simulink model "model_base_bros"  (R2017b)
settings: Solver=FixedStepDiscrete  StartTime=0.0  StopTime=inf  FixedStep=sampleTime  RelTol=1e-3
PostLoadFcn:
  | % load model parameters
  | % pname = fileparts(get_param('model_base_bros','filename'));
  | % run([pname  '\parameters_base_model_bros.m']);
  | parameters_base_model_bros;
  | 
  | % set requested state
  | set_param('model_base_bros/Requested state','Value',num2str(0));
InitFcn:
  | % load model parameters
  | % pname = fileparts(get_param('model_base_bros','filename'));
  | % run([pname  '\parameters_base_model_bros.m']);
  | parameters_base_model_bros;
  | 
  | % set requested state
  | set_param('model_base_bros/Requested state','Value',num2str(0));
StartFcn:
  | % load model parameters
  | % pname = fileparts(get_param('model_base_bros','filename'));
  | % run([pname  '\parameters_base_model_bros.m']);
  | parameters_base_model_bros;
  | 
  | % set requested state
  | set_param('model_base_bros/Requested state','Value',num2str(0));
StopFcn:
  | % switch off data logger (to hopefully avoid corrupt files). TwinCAT doesn't properly switch off the logger when shutting down the model
  | % no idea if this'll work.
  | set_param('model_base_bros/Record data (1 = yes, 0 = no)','Value',num2str(0));
values from neighbouring files (symbols this model uses):
  FFMatrix = -[0 -15; 15 0]    [parameters_base_model_bros.m]
  Lb = 0.07    [parameters_base_model_bros.m]
  Lf = 0.238    [parameters_base_model_bros.m]
  Lu = 0.153    [parameters_base_model_bros.m]
  msin_data_dist1 = [5 11 19 41 59 71 101 137 179 227 0.0358569687947 0.0275584886584 ... (30 elements, 10x3)]    [forcingfunction_data_id.mat]    (also in forcingfunction_data_id_2d_var6_1.mat = [0 0 0 0 0 0 0 0 0 0 0 0 ... (60 elements, 10x6)]; forcingfunction_data_id_2d_var75_nt11.mat = [0 0 0 0 0 0 0 0 0 0 0 0 ... (60 elements, 10x6)]; forcingfunction_data_id_nt10_var6.mat = [5 11 19 41 59 71 101 137 179 227 0.0248424367031 0.01909308)
  msin_data_dist2 = [7 13 23 43 61 73 103 139 181 229 0.0366642780879 0.0272817537998 ... (30 elements, 10x3)]    [forcingfunction_data_id.mat]    (also in forcingfunction_data_id_2d_var6_1.mat = [0 0 0 0 0 0 0 0 0 0 0 0 ... (60 elements, 10x6)]; forcingfunction_data_id_2d_var75_nt11.mat = [0 0 0 0 0 0 0 0 0 0 0 0 ... (60 elements, 10x6)]; forcingfunction_data_id_nt10_var6.mat = [7 13 23 43 61 73 103 139 181 229 0.0254017569884 0.01890135)
  msin_data_target = [2 9 17 27 37 47 0.0347382902327 0.0275101923829 0.0180185190239 0.0110214159229 0.0075682474126 0.00574660779142 ... (18 elements, 6x3)]    [forcingfunction_data_id.mat]    (also in forcingfunction_data_id_2d_var6_1.mat = [5 11 23 37 51 71 101 137 171 226 0.0252651788023 0.01941798; forcingfunction_data_id_2d_var75_nt11.mat = [5 11 23 37 51 71 101 137 173 227 263 0.0282088788597 ... (6; forcingfunction_data_id_nt10_var6.mat = [2 9 17 29 37 47 67 107 149 211 0.0239780224904 0.0189888450; forcingfunction_id_emg.mat = [3 7 13 19 31 0.0450441024419 0.0275859409824 0.015205627144)
  sampleTime = 0.001    [parameters_base_model_bros.m]
  Tm = 81.92    [forcingfunction_data_id_2d_var6_1.mat]    (also in forcingfunction_data_id_2d_var75_nt11.mat; forcingfunction_data_id_nt10_var6.mat; forcingfunction_id_emg.mat = 24)
undefined symbols (not defined in the file or in its folder): BROS1, BROS2, DiscIntNeverNeededParam
libraries: simulink x28, LibraryFM x14, VariousBlocksLibrary x13, simulink_extras x1
(part 2 of 4)

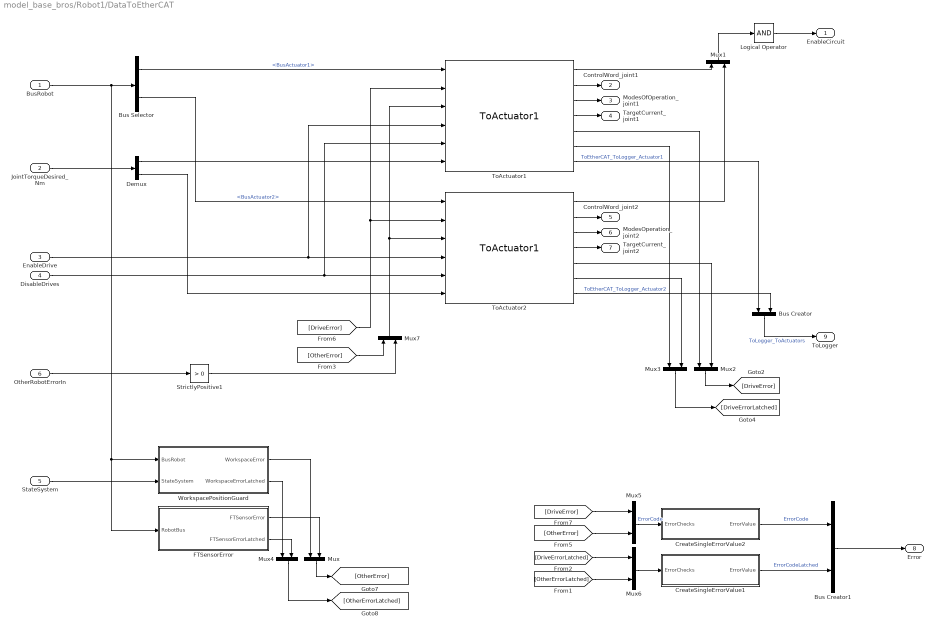
== system model_base_bros/Robot1/DataToEtherCAT ==
  BusRobot : Inport
  JointTorqueDesired_Nm : Inport  Port=2
  EnableDrive : Inport  Port=3
  DisableDrives : Inport  Port=4
  StateSystem : Inport  Port=5
  OtherRobotErrorIn : Inport  Port=6
  Bus Creator : BusCreator  Inputs=2
  Bus Creator1 : BusCreator  Inputs=2
  Bus Selector : BusSelector  OutputSignals=BusActuators.BusActuator1,BusActuators.BusActuator2
  CreateSingleErrorValue1 : Subsystem
  CreateSingleErrorValue2 : Subsystem
  Demux : Demux  Outputs=2
  FTSensorError : Subsystem
  Logical Operator : Logic  Inputs=1  AllPortsSameDT=off  OutDataTypeStr=boolean
  Mux{,1..7} (8 alike) : Mux  Inputs=2
  StrictlyPositive1 : simulink/Logic and Bit Operations/Compare To Zero  relop=>  OutDataTypeStr=boolean
  ToActuator1 : LibraryFM/ToActuator1  ActuatorStruct=RobotStruct.Actuator1
  ToActuator2 : LibraryFM/ToActuator1  ActuatorStruct=RobotStruct.Actuator2
  WorkspacePositionGuard : Subsystem
  EnableCircuit : Outport  OutDataTypeStr=boolean
  ControlWord_joint1 : Outport  Port=2  OutDataTypeStr=uint16
  ModesOfOperation_joint1 : Outport  Port=3  OutDataTypeStr=int8
  TargetCurrent_joint1 : Outport  Port=4  OutDataTypeStr=int16
  ControlWord_joint2 : Outport  Port=5  OutDataTypeStr=uint16
  ModesOperation_joint2 : Outport  Port=6  OutDataTypeStr=int8
  TargetCurrent_joint2 : Outport  Port=7  OutDataTypeStr=int16
  Error : Outport  Port=8
  ToLogger : Outport  Port=9
  wires:
  Bus Creator/1 -> ToLogger/1  "ToLogger_ToActuators"
  ToActuator2/7 -> Bus Creator/2  "ToEtherCAT_ToLogger_Actuator2"
  ToActuator1/7 -> Bus Creator/1  "ToEtherCAT_ToLogger_Actuator1"
  ToActuator1/5 -> Mux2/1
  ToActuator2/5 -> Mux2/2
  Mux2/1 -> [DriveError]
  ToActuator1/6 -> Mux3/1
  ToActuator2/6 -> Mux3/2
  [DriveError] -> ToActuator1/2, ToActuator2/2
  Mux1/1 -> Logical Operator/1
  ToActuator1/1 -> Mux1/1
  ToActuator2/1 -> Mux1/2
  ToActuator1/2 -> ControlWord_joint1/1
  ToActuator1/3 -> ModesOfOperation_joint1/1
  ToActuator2/2 -> ControlWord_joint2/1
  ToActuator1/4 -> TargetCurrent_joint1/1
  ToActuator2/4 -> TargetCurrent_joint2/1
  ToActuator2/3 -> ModesOperation_joint2/1
  Logical Operator/1 -> EnableCircuit/1
  Demux/2 -> ToActuator2/6
  JointTorqueDesired_Nm/1 -> Demux/1
  Demux/1 -> ToActuator1/6
  BusRobot/1 -> WorkspacePositionGuard/1(BusRobot), FTSensorError/1(RobotBus), Bus Selector/1
  Bus Selector/2 -> ToActuator2/1  "<BusActuator2>"
  Bus Selector/1 -> ToActuator1/1  "<BusActuator1>"
  DisableDrives/1 -> ToActuator1/5, ToActuator2/5
  EnableDrive/1 -> ToActuator1/4, ToActuator2/4
  Mux3/1 -> [DriveErrorLatched]
  StateSystem/1 -> WorkspacePositionGuard/2(StateSystem)
  FTSensorError/1(FTSensorError) -> Mux/2
  FTSensorError/2(FTSensorErrorLatched) -> Mux4/2
  WorkspacePositionGuard/1(WorkspaceError) -> Mux/1
  WorkspacePositionGuard/2(WorkspaceErrorLatched) -> Mux4/1
  Mux/1 -> [OtherError]
  Mux4/1 -> [OtherErrorLatched]
  [DriveError] -> Mux5/1
  [OtherError] -> Mux5/2
  CreateSingleErrorValue1/1(ErrorValue) -> Bus Creator1/2  "ErrorCodeLatched"
  [DriveErrorLatched] -> Mux6/1
  [OtherErrorLatched] -> Mux6/2
  Mux6/1 -> CreateSingleErrorValue1/1(ErrorChecks)
  Mux5/1 -> CreateSingleErrorValue2/1(ErrorChecks)  "ErrorCode"
  Bus Creator1/1 -> Error/1
  CreateSingleErrorValue2/1(ErrorValue) -> Bus Creator1/1  "ErrorCode"
  [OtherError] -> Mux7/1
  Mux7/1 -> ToActuator2/3, ToActuator1/3
  OtherRobotErrorIn/1 -> StrictlyPositive1/1
  StrictlyPositive1/1 -> Mux7/2

== system model_base_bros/Robot2/AppendToLoggerBus ==
  BusRobot : Inport
  ToEtherCAT_ToLogger : Inport  Port=2
  Controller_ToLogger : Inport  Port=3
  SystemState : Inport  Port=4
  Bus Creator : BusCreator  Inputs=8
  Bus Selector : BusSelector  OutputSignals=xOpSpace,qJointSpace,BusFTSensor,BusActuators
  Bus Selector1 : BusSelector  OutputSignals=ToEtherCAT_ToLogger_Actuator1,ToEtherCAT_ToLogger_Actuator2
  ToLogger : Outport
  wires:
  Bus Creator/1 -> ToLogger/1  "LoggerBus"
  Bus Selector/4 -> Bus Creator/4  "<BusActuators>"
  Bus Selector/1 -> Bus Creator/1  "<xOpSpace>"
  Bus Selector/3 -> Bus Creator/3  "<BusFTSensor>"
  Bus Selector/2 -> Bus Creator/2  "<qJointSpace>"
  BusRobot/1 -> Bus Selector/1
  ToEtherCAT_ToLogger/1 -> Bus Selector1/1
  Bus Selector1/1 -> Bus Creator/5  "<ToEtherCAT_ToLogger_Actuator1>"
  Bus Selector1/2 -> Bus Creator/6  "<ToEtherCAT_ToLogger_Actuator2>"
  Controller_ToLogger/1 -> Bus Creator/7
  SystemState/1 -> Bus Creator/8  "SystemState"

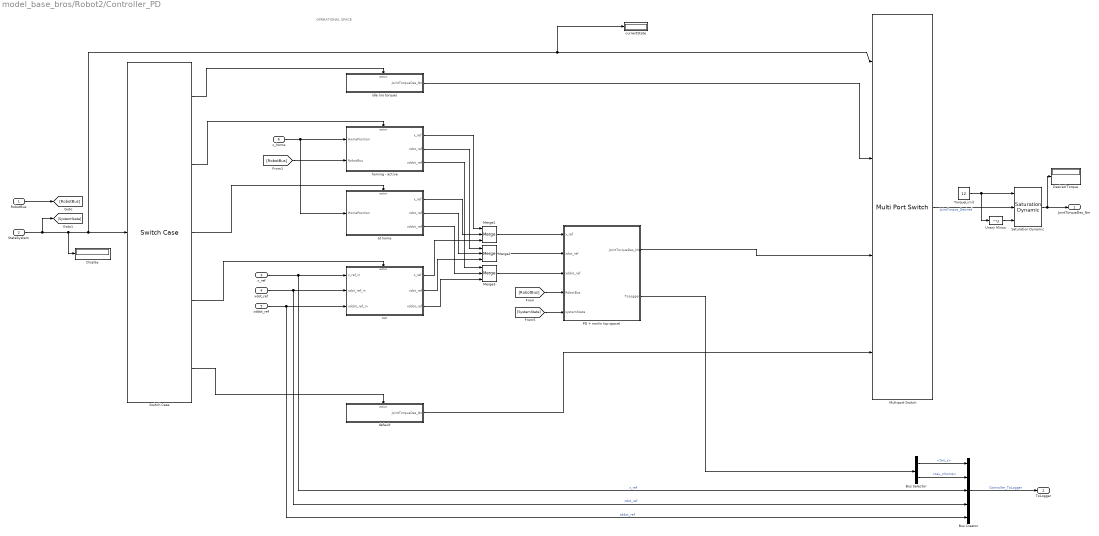
== system model_base_bros/Robot2/Controller_PD ==
  note: OPERATIONAL SPACE
  RobotBus : Inport
  StateSystem : Inport  Port=2
  x_ref : Inport  Port=3
  xdot_ref : Inport  Port=4
  xddot_ref : Inport  Port=5
  x_home : Inport  Port=6
  Bus Creator : BusCreator  Inputs=5
  Bus Selector : BusSelector  OutputSignals=tau_y,tau_nlcomp
  Desired Torque : Display
  Display : Display
  Merge1 : Merge  Inputs=3  InitialOutput=[0;0]
  Merge2 : Merge  Inputs=3  InitialOutput=[0;0]
  Merge3 : Merge  Inputs=3  InitialOutput=[0;0]
  Multiport Switch : MultiPortSwitch  DataPortOrder=Specify indices  Inputs=4  DataPortIndices={[0,1,2,201,299,301],[302,399,4]}  DataPortForDefault=Additional data port
  PD + nonlin (op space) : Subsystem
  Saturation Dynamic : simulink/Discontinuities/Saturation Dynamic  OutMin=[]  OutMax=[]  OutDataTypeStr=Inherit: Same as second input  OutDataType=fixdt(1, 16)  OutScaling=2^-10  DoSatur=off
  Switch Case : SwitchCase  CaseConditions={[0,1,2,201,299,301],302, 399,[4]}
  TorqueLimit : Constant  Value=12
  Unary Minus : UnaryMinus
  at home : Subsystem
  currentState : Display
  default : Subsystem  TreatAsAtomicUnit=on
  homing - active : Subsystem
  idle (no torque) : Subsystem  TreatAsAtomicUnit=on
  run : Subsystem
  JointTorqueDes_Nm : Outport
  ToLogger : Outport  Port=2
  wires:
  [SystemState] -> PD + nonlin (op space)/5(systemState)
  xddot_ref/1 -> Bus Creator/5, run/3(xddot_ref_in)  "xddot_ref"
  xdot_ref/1 -> Bus Creator/4, run/2(xdot_ref_in)  "xdot_ref"
  x_ref/1 -> Bus Creator/3, run/1(x_ref_in)  "x_ref"
  [RobotBus] -> PD + nonlin (op space)/4(RobotBus)
  RobotBus/1 -> [RobotBus]
  Merge3/1 -> PD + nonlin (op space)/3(xddot_ref)
  Merge2/1 -> PD + nonlin (op space)/2(xdot_ref)
  Merge1/1 -> PD + nonlin (op space)/1(x_ref)
  idle (no torque)/1(JointTorqueDes_Nm) -> Multiport Switch/2
  Switch Case/2 -> homing - active/Action
  Switch Case/1 -> idle (no torque)/Action
  default/1(JointTorqueDes_Nm) -> Multiport Switch/4
  Switch Case/5 -> default/Action
  Saturation Dynamic/1 -> Desired Torque/1, JointTorqueDes_Nm/1
  Switch Case/3 -> at home/Action
  homing - active/1(x_ref) -> Merge1/1
  run/1(x_ref) -> Merge1/3
  StateSystem/1 -> Display/1, Multiport Switch/1, currentState/1, Switch Case/1, [SystemState]
  run/2(xdot_ref) -> Merge2/3
  run/3(xddot_ref) -> Merge3/3
  homing - active/2(xdot_ref) -> Merge2/1
  homing - active/3(xddot_ref) -> Merge3/1
  Multiport Switch/1 -> Saturation Dynamic/2  "JointTorque_Desired"
  PD + nonlin (op space)/2(ToLogger) -> Bus Selector/1
  x_home/1 -> at home/1(HomePosition), homing - active/1(HomePosition)
  Bus Creator/1 -> ToLogger/1  "Controller_ToLogger"
  Bus Selector/1 -> Bus Creator/1  "<tau_y>"
  Bus Selector/2 -> Bus Creator/2  "<tau_nlcomp>"
  TorqueLimit/1 -> Unary Minus/1, Saturation Dynamic/1
  Unary Minus/1 -> Saturation Dynamic/3
  [RobotBus] -> homing - active/2(RobotBus)
  at home/1(x_ref) -> Merge1/2
  at home/2(xdot_ref) -> Merge2/2
  at home/3(xddot_ref) -> Merge3/2
  Switch Case/4 -> run/Action
  PD + nonlin (op space)/1(JointTorqueDes_Nm) -> Multiport Switch/3

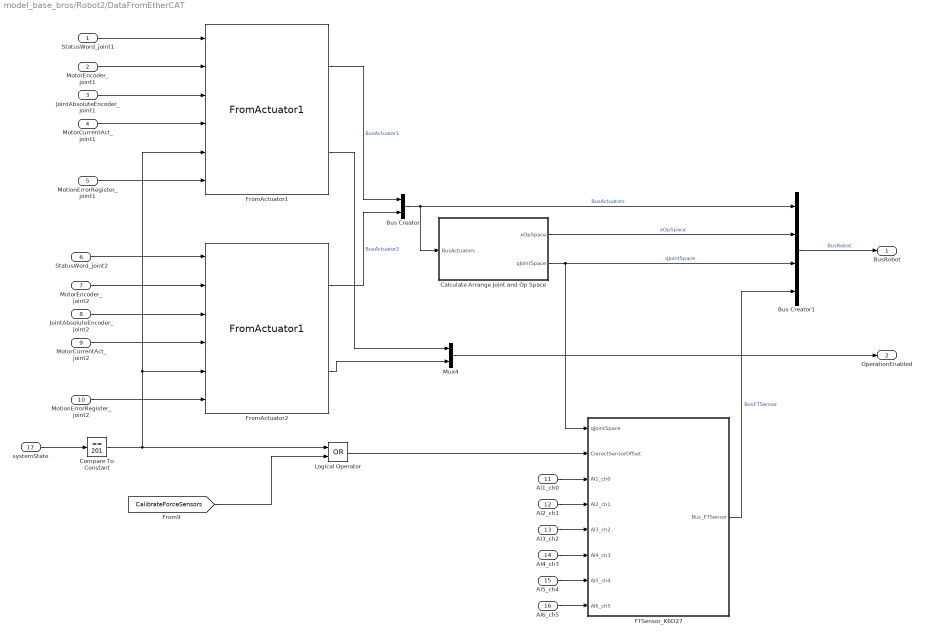
== system model_base_bros/Robot2/DataFromEtherCAT ==
  StatusWord_joint1 : Inport
  MotorEncoder_joint1 : Inport  Port=2
  JointAbsoluteEncoder_joint1 : Inport  Port=3
  MotorCurrentAct_joint1 : Inport  Port=4
  MotionErrorRegister_joint1 : Inport  Port=5  OutDataTypeStr=uint16
  StatusWord_joint2 : Inport  Port=6
  MotorEncoder_joint2 : Inport  Port=7
  "JointAbsoluteEncoder_joint2 " : Inport  Port=8
  MotorCurrentAct_joint2 : Inport  Port=9
  MotionErrorRegister_joint2 : Inport  Port=10  OutDataTypeStr=uint16
  AI1_ch0 : Inport  Port=11
  AI2_ch1 : Inport  Port=12
  AI3_ch2 : Inport  Port=13
  AI4_ch3 : Inport  Port=14
  AI5_ch4 : Inport  Port=15
  AI6_ch5 : Inport  Port=16
  systemState : Inport  Port=17
  Bus Creator : BusCreator  Inputs=2
  Bus Creator1 : BusCreator  Inputs=4
  Calculate Arrange Joint and Op Space : Subsystem
  Compare To Constant : simulink/Logic and Bit Operations/Compare To Constant  relop===  const=201  OutDataTypeStr=boolean
  FTSensor_K6D27 : Subsystem  mask{FTSensorStruct=RobotStruct.FTSensor}
      mask prompts: FTSensorStruct "Struct for force torque sensor"
  FromActuator1 : LibraryFM/FromActuator1  ActuatorStruct=RobotStruct.Actuator1
  FromActuator2 : LibraryFM/FromActuator1  ActuatorStruct=RobotStruct.Actuator2
  Logical Operator : Logic  Operator=OR  AllPortsSameDT=off  OutDataTypeStr=boolean
  Mux4 : Mux  Inputs=2
  BusRobot : Outport
  OperationEnabled : Outport  Port=2
  wires:
  FTSensor_K6D27/1(Bus_FTSensor) -> Bus Creator1/4  "BusFTSensor"
  FromActuator1/1 -> Bus Creator/1  "BusActuator1"
  FromActuator2/1 -> Bus Creator/2  "BusActuator2"
  FromActuator1/2 -> Mux4/1
  Mux4/1 -> OperationEnabled/1
  FromActuator2/2 -> Mux4/2
  MotorEncoder_joint1/1 -> FromActuator1/2
  StatusWord_joint1/1 -> FromActuator1/1
  JointAbsoluteEncoder_joint1/1 -> FromActuator1/3
  MotorCurrentAct_joint1/1 -> FromActuator1/4
  MotorEncoder_joint2/1 -> FromActuator2/2
  StatusWord_joint2/1 -> FromActuator2/1
  "JointAbsoluteEncoder_joint2 "/1 -> FromActuator2/3
  MotorCurrentAct_joint2/1 -> FromActuator2/4
  Bus Creator/1 -> Calculate Arrange Joint and Op Space/1(BusActuators), Bus Creator1/1  "BusActuators"
  Bus Creator1/1 -> BusRobot/1  "BusRobot"
  Calculate Arrange Joint and Op Space/2(qJointSpace) -> FTSensor_K6D27/1(qJointSpace), Bus Creator1/3  "qJointSpace"
  systemState/1 -> Compare To Constant/1
  AI1_ch0/1 -> FTSensor_K6D27/3(AI1_ch0)
  AI2_ch1/1 -> FTSensor_K6D27/4(AI2_ch1)
  AI3_ch2/1 -> FTSensor_K6D27/5(AI3_ch2)
  AI4_ch3/1 -> FTSensor_K6D27/6(AI4_ch3)
  AI5_ch4/1 -> FTSensor_K6D27/7(AI5_ch4)
  AI6_ch5/1 -> FTSensor_K6D27/8(AI6_ch5)
  Compare To Constant/1 -> Logical Operator/1, FromActuator1/5, FromActuator2/5
  Calculate Arrange Joint and Op Space/1(xOpSpace) -> Bus Creator1/2  "xOpSpace"
  [CalibrateForceSensors] -> Logical Operator/2
  Logical Operator/1 -> FTSensor_K6D27/2(CorrectSensorOffset)
  MotionErrorRegister_joint1/1 -> FromActuator1/6
  MotionErrorRegister_joint2/1 -> FromActuator2/6

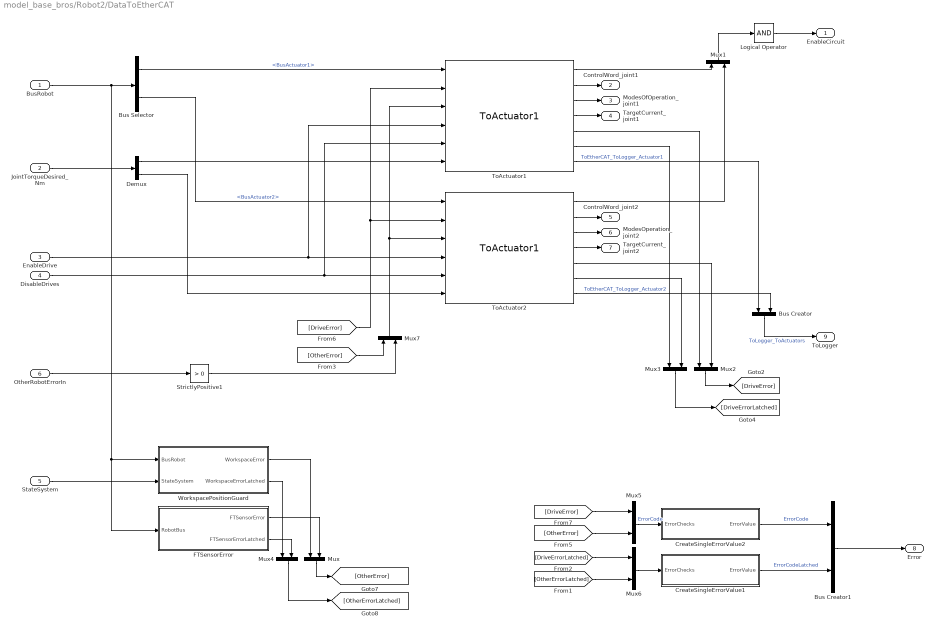
== system model_base_bros/Robot2/DataToEtherCAT ==
  BusRobot : Inport
  JointTorqueDesired_Nm : Inport  Port=2
  EnableDrive : Inport  Port=3
  DisableDrives : Inport  Port=4
  StateSystem : Inport  Port=5
  OtherRobotErrorIn : Inport  Port=6
  Bus Creator : BusCreator  Inputs=2
  Bus Creator1 : BusCreator  Inputs=2
  Bus Selector : BusSelector  OutputSignals=BusActuators.BusActuator1,BusActuators.BusActuator2
  CreateSingleErrorValue1 : Subsystem
  CreateSingleErrorValue2 : Subsystem
  Demux : Demux  Outputs=2
  FTSensorError : Subsystem
  Logical Operator : Logic  Inputs=1  AllPortsSameDT=off  OutDataTypeStr=boolean
  Mux{,1..7} (8 alike) : Mux  Inputs=2
  StrictlyPositive1 : simulink/Logic and Bit Operations/Compare To Zero  relop=>  OutDataTypeStr=boolean
  ToActuator1 : LibraryFM/ToActuator1  ActuatorStruct=RobotStruct.Actuator1
  ToActuator2 : LibraryFM/ToActuator1  ActuatorStruct=RobotStruct.Actuator2
  WorkspacePositionGuard : Subsystem
  EnableCircuit : Outport  OutDataTypeStr=boolean
  ControlWord_joint1 : Outport  Port=2  OutDataTypeStr=uint16
  ModesOfOperation_joint1 : Outport  Port=3  OutDataTypeStr=int8
  TargetCurrent_joint1 : Outport  Port=4  OutDataTypeStr=int16
  ControlWord_joint2 : Outport  Port=5  OutDataTypeStr=uint16
  ModesOperation_joint2 : Outport  Port=6  OutDataTypeStr=int8
  TargetCurrent_joint2 : Outport  Port=7  OutDataTypeStr=int16
  Error : Outport  Port=8
  ToLogger : Outport  Port=9
  wires:
  Bus Creator/1 -> ToLogger/1  "ToLogger_ToActuators"
  ToActuator2/7 -> Bus Creator/2  "ToEtherCAT_ToLogger_Actuator2"
  ToActuator1/7 -> Bus Creator/1  "ToEtherCAT_ToLogger_Actuator1"
  ToActuator1/5 -> Mux2/1
  ToActuator2/5 -> Mux2/2
  Mux2/1 -> [DriveError]
  ToActuator1/6 -> Mux3/1
  ToActuator2/6 -> Mux3/2
  [DriveError] -> ToActuator1/2, ToActuator2/2
  Mux1/1 -> Logical Operator/1
  ToActuator1/1 -> Mux1/1
  ToActuator2/1 -> Mux1/2
  ToActuator1/2 -> ControlWord_joint1/1
  ToActuator1/3 -> ModesOfOperation_joint1/1
  ToActuator2/2 -> ControlWord_joint2/1
  ToActuator1/4 -> TargetCurrent_joint1/1
  ToActuator2/4 -> TargetCurrent_joint2/1
  ToActuator2/3 -> ModesOperation_joint2/1
  Logical Operator/1 -> EnableCircuit/1
  Demux/2 -> ToActuator2/6
  JointTorqueDesired_Nm/1 -> Demux/1
  Demux/1 -> ToActuator1/6
  BusRobot/1 -> WorkspacePositionGuard/1(BusRobot), FTSensorError/1(RobotBus), Bus Selector/1
  Bus Selector/2 -> ToActuator2/1  "<BusActuator2>"
  Bus Selector/1 -> ToActuator1/1  "<BusActuator1>"
  DisableDrives/1 -> ToActuator1/5, ToActuator2/5
  EnableDrive/1 -> ToActuator1/4, ToActuator2/4
  Mux3/1 -> [DriveErrorLatched]
  StateSystem/1 -> WorkspacePositionGuard/2(StateSystem)
  FTSensorError/1(FTSensorError) -> Mux/2
  FTSensorError/2(FTSensorErrorLatched) -> Mux4/2
  WorkspacePositionGuard/1(WorkspaceError) -> Mux/1
  WorkspacePositionGuard/2(WorkspaceErrorLatched) -> Mux4/1
  Mux/1 -> [OtherError]
  Mux4/1 -> [OtherErrorLatched]
  [DriveError] -> Mux5/1
  [OtherError] -> Mux5/2
  CreateSingleErrorValue1/1(ErrorValue) -> Bus Creator1/2  "ErrorCodeLatched"
  [DriveErrorLatched] -> Mux6/1
  [OtherErrorLatched] -> Mux6/2
  Mux6/1 -> CreateSingleErrorValue1/1(ErrorChecks)
  Mux5/1 -> CreateSingleErrorValue2/1(ErrorChecks)  "ErrorCode"
  Bus Creator1/1 -> Error/1
  CreateSingleErrorValue2/1(ErrorValue) -> Bus Creator1/1  "ErrorCode"
  [OtherError] -> Mux7/1
  Mux7/1 -> ToActuator2/3, ToActuator1/3
  OtherRobotErrorIn/1 -> StrictlyPositive1/1
  StrictlyPositive1/1 -> Mux7/2

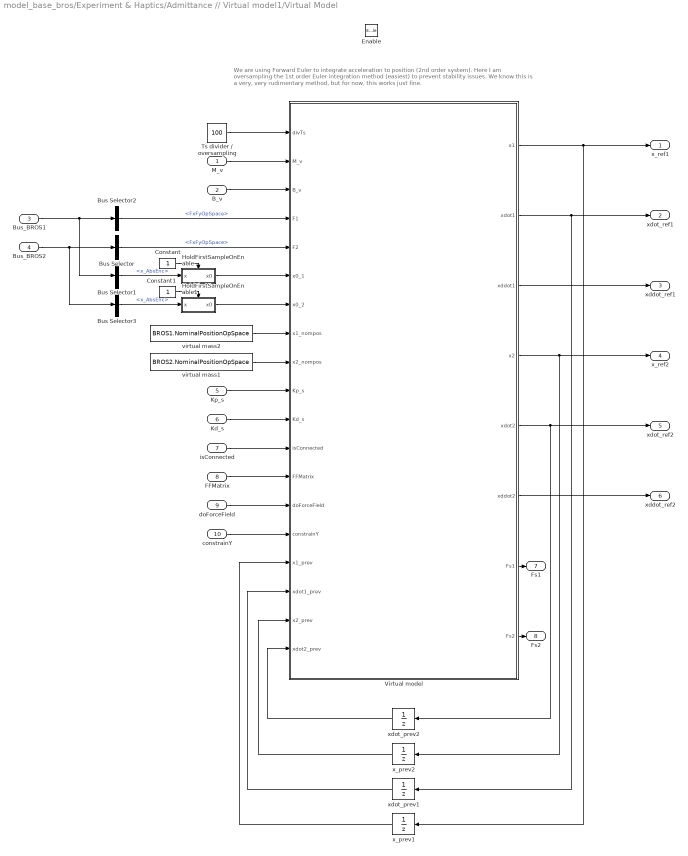
== system model_base_bros/Experiment & Haptics/Admittance // Virtual model1/Virtual Model ==
  note: We are using Forward Euler to integrate acceleration to position (2nd order system).
      | Here I am oversampling the 1st order Euler integration method (easiest) to prevent stability issues.
      | We know this is a very, very rudimentary method, but for now, this works just fine.
  M_v : Inport
  B_v : Inport  Port=2
  Bus_BROS1 : Inport  Port=3
  Bus_BROS2 : Inport  Port=4
  Kp_s : Inport  Port=5
  Kd_s : Inport  Port=6
  isConnected : Inport  Port=7
  FFMatrix : Inport  Port=8
  doForceField : Inport  Port=9
  constrainY : Inport  Port=10
  Enable : EnablePort  StatesWhenEnabling=reset
  Bus Selector : BusSelector  OutputSignals=BusFTSensor.FxFyOpSpace
  Bus Selector1 : BusSelector  OutputSignals=xOpSpace.x_AbsEnc
  Bus Selector2 : BusSelector  OutputSignals=BusFTSensor.FxFyOpSpace
  Bus Selector3 : BusSelector  OutputSignals=xOpSpace.x_AbsEnc
  Constant : Constant
  Constant1 : Constant
  HoldFirstSampleOnEnable : Subsystem
  HoldFirstSampleOnEnable1 : Subsystem
  Ts divider / oversampling : Constant  Value=100
  Virtual model : MATLAB Function  TreatAsAtomicUnit=on
  virtual mass1 : Constant  Value=BROS2.NominalPositionOpSpace
  virtual mass2 : Constant  Value=BROS1.NominalPositionOpSpace
  x_prev1 : UnitDelay  SampleTime=-1
  x_prev2 : UnitDelay  SampleTime=-1
  "xdot_prev1 " : UnitDelay  SampleTime=-1
  xdot_prev2 : UnitDelay  SampleTime=-1
  x_ref1 : Outport
  xdot_ref1 : Outport  Port=2
  xddot_ref1 : Outport  Port=3
  x_ref2 : Outport  Port=4
  xdot_ref2 : Outport  Port=5
  xddot_ref2 : Outport  Port=6
  Fs1 : Outport  Port=7
  Fs2 : Outport  Port=8
  wires:
  Constant/1 -> HoldFirstSampleOnEnable/Enable
  Bus Selector1/1 -> HoldFirstSampleOnEnable/1(x)  "<x_AbsEnc>"
  Bus Selector/1 -> Virtual model/5(F2)  "<FxFyOpSpace>"
  Virtual model/3(xddot1) -> xddot_ref1/1
  Virtual model/2(xdot1) -> xdot_ref1/1, "xdot_prev1 "/1
  HoldFirstSampleOnEnable1/1(x0) -> Virtual model/7(x0_2)
  Virtual model/4(x2) -> x_prev2/1, x_ref2/1
  x_prev1/1 -> Virtual model/16(x1_prev)
  virtual mass1/1 -> Virtual model/9(x2_nompos)
  virtual mass2/1 -> Virtual model/8(x1_nompos)
  Bus Selector2/1 -> Virtual model/4(F1)  "<FxFyOpSpace>"
  "xdot_prev1 "/1 -> Virtual model/17(xdot1_prev)
  isConnected/1 -> Virtual model/12(isConnected)
  x_prev2/1 -> Virtual model/18(x2_prev)
  Constant1/1 -> HoldFirstSampleOnEnable1/Enable
  Bus Selector3/1 -> HoldFirstSampleOnEnable1/1(x)  "<x_AbsEnc>"
  Kp_s/1 -> Virtual model/10(Kp_s)
  Kd_s/1 -> Virtual model/11(Kd_s)
  xdot_prev2/1 -> Virtual model/19(xdot2_prev)
  B_v/1 -> Virtual model/3(B_v)
  Bus_BROS1/1 -> Bus Selector2/1, Bus Selector1/1
  M_v/1 -> Virtual model/2(M_v)
  Bus_BROS2/1 -> Bus Selector3/1, Bus Selector/1
  HoldFirstSampleOnEnable/1(x0) -> Virtual model/6(x0_1)
  Virtual model/6(xddot2) -> xddot_ref2/1
  Virtual model/1(x1) -> x_ref1/1, x_prev1/1
  Virtual model/5(xdot2) -> xdot_prev2/1, xdot_ref2/1
  Ts divider / oversampling/1 -> Virtual model/1(divTs)
  doForceField/1 -> Virtual model/14(doForceField)
  FFMatrix/1 -> Virtual model/13(FFMatrix)
  Virtual model/7(Fs1) -> Fs1/1
  Virtual model/8(Fs2) -> Fs2/1
  constrainY/1 -> Virtual model/15(constrainY)

== system model_base_bros/Experiment & Haptics/Trial Logic/StopWatch ==
  Enable : EnablePort  StatesWhenEnabling=reset
  Counter Free-Running : simulink/Sources/Counter Free-Running  NumBits=32  tsamp=-1
  Data Type Conversion : DataTypeConversion  OutDataTypeStr=double
  sample time : Gain  Gain=sampleTime
  trialTime : Outport
  wires:
  sample time/1 -> trialTime/1
  Data Type Conversion/1 -> sample time/1
  Counter Free-Running/1 -> Data Type Conversion/1

== system model_base_bros/Robot1/Controller_PD/PD + nonlin (op space) ==
  x_ref : Inport
  xdot_ref : Inport  Port=2
  xddot_ref : Inport  Port=3
  RobotBus : Inport  Port=4
  systemState : Inport  Port=5
  Bus Creator : BusCreator  Inputs=2
  Bus Selector : BusSelector  OutputSignals=xOpSpace.x,xOpSpace.xdot,xOpSpace.x_AbsEnc,xOpSpace.xdot_AbsEnc,xOpSpace.J,xOpSpace.Jdot,qJointSpace.qdot_IncEnc
  DesiredTorque_PID : Display
  Gain : Gain  Gain=0
  Kd : Gain  Gain=15
  Kd1 : Gain  Gain=0
  Kd2 : Gain  Gain=5
  Kp : Gain  Gain=1500
  Sum{,2,4..5} (4 alike) : Sum  Inputs=|+-
  Sum1 : Sum  Inputs=|++
  Sum3 : Sum  Inputs=++++
  Terminator : Terminator
  Terminator1 : Terminator
  invJ1 : MATLAB Function  TreatAsAtomicUnit=on
  nonlinear compensation : MATLAB Function  TreatAsAtomicUnit=on
  JointTorqueDes_Nm : Outport
  ToLogger : Outport  Port=2
  wires:
  nonlinear compensation/1(tau) -> Gain/1, Bus Creator/2  "tau_nlcomp"
  invJ1/1(y) -> Sum1/1, Bus Creator/1  "tau_y"
  Bus Selector/1 -> Sum/2  "<x>"
  x_ref/1 -> Sum/1, Sum4/1  "q_ref"
  Sum/1 -> Kp/1  "e_p"
  xdot_ref/1 -> Sum5/1, Sum2/1  "qdot_ref"
  Sum2/1 -> Kd/1  "e_d"
  Sum1/1 -> JointTorqueDes_Nm/1, DesiredTorque_PID/1
  systemState/1 -> Terminator/1
  Bus Creator/1 -> ToLogger/1  "ToLoggerPD"
  Gain/1 -> Sum1/2
  Bus Selector/2 -> Sum2/2  "<xdot>"
  Bus Selector/6 -> nonlinear compensation/2(Jdot)  "<Jdot>"
  Bus Selector/5 -> nonlinear compensation/1(J), invJ1/2(J)  "<J>"
  RobotBus/1 -> Bus Selector/1
  Sum4/1 -> Kd1/1
  Sum5/1 -> Kd2/1
  xddot_ref/1 -> Terminator1/1  "qddot_ref"
  Bus Selector/3 -> Sum4/2  "<x_AbsEnc>"
  Bus Selector/4 -> Sum5/2  "<xdot_AbsEnc>"
  Kd/1 -> Sum3/2
  Kp/1 -> Sum3/1
  Sum3/1 -> invJ1/1(x)
  Kd1/1 -> Sum3/3
  Kd2/1 -> Sum3/4
  Bus Selector/7 -> nonlinear compensation/3(qdot)  "<qdot_IncEnc>"

== system model_base_bros/Robot1/Controller_PD/at home ==
  note: The velocity and acceleration references are set to [0;0] for stability.
  HomePosition : Inport
  Action Port : ActionPort  InitializeStates=reset  ActionType=case
  Constant : Constant
  Constant2 : Constant  Value=[0;0]
  Constant4 : Constant  Value=[0;0]
  HoldFirstSampleOnEnable : Subsystem
  x_ref : Outport  InitialOutput=[0;0]
  xdot_ref : Outport  Port=2  InitialOutput=[0;0]
  xddot_ref : Outport  Port=3  InitialOutput=[0;0]
  wires:
  Constant2/1 -> xdot_ref/1
  HoldFirstSampleOnEnable/1(x0) -> x_ref/1
  Constant4/1 -> xddot_ref/1
  Constant/1 -> HoldFirstSampleOnEnable/Enable
  HomePosition/1 -> HoldFirstSampleOnEnable/1(x)

== system model_base_bros/Robot1/Controller_PD/default ==
  Action Port : ActionPort  InitializeStates=reset  ActionType=default
  Constant3 : Constant  Value=[0;0]
  JointTorqueDes_Nm : Outport  InitialOutput=[0;0]
  wires:
  Constant3/1 -> JointTorqueDes_Nm/1

== system model_base_bros/Robot1/Controller_PD/homing - active ==
  note: The velocity and acceleration references are set to [0;0] for stability.
  HomePosition : Inport
  RobotBus : Inport  Port=2
  Action Port : ActionPort  InitializeStates=reset  ActionType=case
  Bus Selector : BusSelector  OutputSignals=xOpSpace.x
  Constant1 : Constant
  Constant2 : Constant  Value=[0;0]
  Constant4 : Constant  Value=[0;0]
  CrossFade : VariousBlocksLibrary/Various/CrossFade
  Cycloid : VariousBlocksLibrary/Various/Cycloid
  Rate Limiter : RateLimiter  RisingSlewLimit=0.1  FallingSlewLimit=-0.2  SampleTimeMode=inherited
  x_ref : Outport  InitialOutput=[0;0]
  xdot_ref : Outport  Port=2  InitialOutput=[0;0]
  xddot_ref : Outport  Port=3  InitialOutput=[0;0]
  wires:
  Constant2/1 -> xdot_ref/1
  Bus Selector/1 -> CrossFade/1  "<x>"
  RobotBus/1 -> Bus Selector/1
  HomePosition/1 -> CrossFade/2
  Cycloid/1 -> CrossFade/3
  Rate Limiter/1 -> Cycloid/1
  Constant1/1 -> Rate Limiter/1
  CrossFade/1 -> x_ref/1
  Constant4/1 -> xddot_ref/1

== system model_base_bros/Robot1/Controller_PD/idle (no torque) ==
  Action Port : ActionPort  InitializeStates=reset  ActionType=case
  Constant3 : Constant  Value=[0;0]
  JointTorqueDes_Nm : Outport  InitialOutput=[0;0]
  wires:
  Constant3/1 -> JointTorqueDes_Nm/1

== system model_base_bros/Robot1/Controller_PD/run ==
  x_ref_in : Inport
  xdot_ref_in : Inport  Port=2
  xddot_ref_in : Inport  Port=3
  Action Port : ActionPort  InitializeStates=reset  ActionType=case
  x_ref : Outport  InitialOutput=[0;0]
  xdot_ref : Outport  Port=2  InitialOutput=[0;0]
  xddot_ref : Outport  Port=3  InitialOutput=[0;0]
  wires:
  xdot_ref_in/1 -> xdot_ref/1
  xddot_ref_in/1 -> xddot_ref/1
  x_ref_in/1 -> x_ref/1

== system model_base_bros/Robot1/DataFromEtherCAT/Calculate Arrange Joint and Op Space ==
  note: Here all angles of the parallel mechanism are calculated
      | based on the endpoint position, though this may still lead to incorrect
      | estimations of the internal angles (e.g. it is possible that on of the elbows
      | has gone through a singular position already). So perhaps I should also include
      | a different way of calculating the internal angles
  BusActuators : Inport
  Bus Creator1 : BusCreator  Inputs=9
  Bus Creator2 : BusCreator  Inputs=6
  Bus Selector1 : BusSelector  OutputSignals=BusActuator1.JointPosition_AbsEnc_rad,BusActuator2.JointPosition_AbsEnc_rad,BusActuator1.JointVelocity_AbsEnc_rads,BusActuator2.JointVelocity_AbsEnc_rads
  Bus Selector2 : BusSelector  OutputSignals=BusActuator1.JointPosition_IncEnc_rad,BusActuator2.JointPosition_IncEnc_rad,BusActuator1.JointVelocity_IncEnc_rads,BusActuator2.JointVelocity_IncEnc_rads
  Bus Selector3 : BusSelector  OutputSignals=BusActuator1.JointTorque_Act_Nm,BusActuator2.JointTorque_Act_Nm
  Condition number : MATLAB Function  TreatAsAtomicUnit=on
  Ground : Ground
  Ground1 : Ground
  IK all joints : MATLAB Function  TreatAsAtomicUnit=on
  Mux{,1..4} (5 alike) : Mux  Inputs=2
  Terminator1 : Terminator
  Terminator2 : Terminator
  forward kinematics : Subsystem
  forward kinematics1 : Subsystem
  xOpSpace : Outport
  qJointSpace : Outport  Port=2
  wires:
  forward kinematics/5(Jdot) -> Bus Creator1/4  "Jdot"
  forward kinematics/3(xddot) -> Terminator1/1
  forward kinematics/2(xdot) -> Bus Creator1/2  "xdot"
  forward kinematics/1(x) -> IK all joints/1(x), Bus Creator1/1  "x"
  Bus Creator1/1 -> xOpSpace/1  "xOpSpace"
  forward kinematics/4(J) -> Condition number/1(J), Bus Creator1/3  "J"
  Ground/1 -> forward kinematics/3(JointAcceleration_rads2)
  Bus Creator2/1 -> qJointSpace/1  "qJointSpace"
  BusActuators/1 -> Bus Selector1/1, Bus Selector3/1, Bus Selector2/1
  Bus Selector2/1 -> Mux/1  "<JointPosition_IncEnc_rad>"
  Bus Selector2/2 -> Mux/2  "<JointPosition_IncEnc_rad>"
  Bus Selector2/3 -> Mux1/1  "<JointVelocity_IncEnc_rads>"
  Bus Selector2/4 -> Mux1/2  "<JointVelocity_IncEnc_rads>"
  Mux1/1 -> Bus Creator2/3, forward kinematics/2(JointVelocity_rads)  "qdot_IncEnc"
  Mux/1 -> forward kinematics/1(JointPosition_rad), Bus Creator2/2  "q_IncEnc"
  IK all joints/1(q_all) -> Bus Creator2/6  "q_all"
  Condition number/1(C) -> Bus Creator1/5  "conditioning"
  Bus Selector1/4 -> Mux3/2  "<JointVelocity_AbsEnc_rads>"
  Bus Selector1/3 -> Mux3/1  "<JointVelocity_AbsEnc_rads>"
  Bus Selector1/2 -> Mux2/2  "<JointPosition_AbsEnc_rad>"
  Bus Selector1/1 -> Mux2/1  "<JointPosition_AbsEnc_rad>"
  forward kinematics1/3(xddot) -> Terminator2/1
  Ground1/1 -> forward kinematics1/3(JointAcceleration_rads2)
  Mux2/1 -> Bus Creator2/4, forward kinematics1/1(JointPosition_rad)  "q_AbsEnc"
  Mux3/1 -> Bus Creator2/5, forward kinematics1/2(JointVelocity_rads)  "qdot_AbsEnc"
  forward kinematics1/2(xdot) -> Bus Creator1/7  "xdot_AbsEnc"
  forward kinematics1/1(x) -> Bus Creator1/6  "x_AbsEnc"
  forward kinematics1/4(J) -> Bus Creator1/8  "J_AbsEnc"
  forward kinematics1/5(Jdot) -> Bus Creator1/9  "Jdot_AbsEnc"
  Bus Selector3/1 -> Mux4/1  "<JointTorque_Act_Nm>"
  Bus Selector3/2 -> Mux4/2  "<JointTorque_Act_Nm>"
  Mux4/1 -> Bus Creator2/1  "JointTorque_Nm"

== system model_base_bros/Robot1/DataFromEtherCAT/FTSensor_K6D27 ==
  qJointSpace : Inport
  CorrectSensorOffset : Inport  Port=2
  AI1_ch0 : Inport  Port=3
  AI2_ch1 : Inport  Port=4
  AI3_ch2 : Inport  Port=5
  AI4_ch3 : Inport  Port=6
  AI5_ch4 : Inport  Port=7
  AI6_ch5 : Inport  Port=8
  Bus Creator : BusCreator  Inputs=3
  Bus Selector : BusSelector  OutputSignals=q_all
  Constant : Constant  Value=FTSensorStruct.TransformationMatrixSide
  CorrectOffset : MATLAB Function  TreatAsAtomicUnit=on
  Data Type Conversion{,1..5} (6 alike) : DataTypeConversion  OutDataTypeStr=double
  Detect Increase : simulink/Logic and Bit Operations/Detect Increase  vinit=0.0  InputProcessing=Inherited  OutDataTypeStr=boolean
  Mux : Mux  Inputs=6
  Selector : Selector  InputPortWidth=6  IndexOptions=Index vector (dialog)  Indices=[1 2]  OutputSizes=1
  SensorToOperationalSpace : MATLAB Function  TreatAsAtomicUnit=on
  Terminator : Terminator
  force (op space) : Display
  force (sensor space) : Display
  spikefilter : Subsystem
  Bus_FTSensor : Outport
  wires:
  Constant/1 -> SensorToOperationalSpace/3(transmatside)
  Bus Creator/1 -> Bus_FTSensor/1  "BusFTSensor"
  SensorToOperationalSpace/1(FTOpSpace) -> Selector/1, force (op space)/1, Bus Creator/1  "ForcesOpSpace"
  Data Type Conversion5/1 -> Mux/6
  Data Type Conversion4/1 -> Mux/5
  Data Type Conversion3/1 -> Mux/4
  Data Type Conversion2/1 -> Mux/3
  Data Type Conversion1/1 -> Mux/2
  Data Type Conversion/1 -> Mux/1
  CorrectOffset/1(u_out) -> spikefilter/1(in)  "ForcesSensorSpace"
  CorrectOffset/2(corrected) -> Terminator/1
  AI3_ch2/1 -> Data Type Conversion2/1
  AI4_ch3/1 -> Data Type Conversion3/1
  AI5_ch4/1 -> Data Type Conversion4/1
  AI6_ch5/1 -> Data Type Conversion5/1
  Detect Increase/1 -> CorrectOffset/2(reset)
  CorrectSensorOffset/1 -> Detect Increase/1
  Mux/1 -> CorrectOffset/1(u_in)
  AI1_ch0/1 -> Data Type Conversion/1
  AI2_ch1/1 -> Data Type Conversion1/1
  qJointSpace/1 -> Bus Selector/1
  Bus Selector/1 -> SensorToOperationalSpace/1(q_all)  "<q_all>"
  Selector/1 -> Bus Creator/2  "FxFyOpSpace"
  spikefilter/1(out) -> SensorToOperationalSpace/2(Fs), Bus Creator/3, force (sensor space)/1  "ForcesSensorSpace"

== system model_base_bros/Robot1/DataToEtherCAT/CreateSingleErrorValue1 ==
  ErrorChecks : Inport
  Data Type Conversion1 : DataTypeConversion  OutDataTypeStr=double
  ErrorToPower2 : MATLAB Function  TreatAsAtomicUnit=on
  ErrorValue : Outport
  wires:
  Data Type Conversion1/1 -> ErrorToPower2/1(u)
  ErrorChecks/1 -> Data Type Conversion1/1
  ErrorToPower2/1(e) -> ErrorValue/1

== system model_base_bros/Robot1/DataToEtherCAT/CreateSingleErrorValue2 ==
  ErrorChecks : Inport
  Data Type Conversion1 : DataTypeConversion  OutDataTypeStr=double
  ErrorToPower2 : MATLAB Function  TreatAsAtomicUnit=on
  ErrorValue : Outport
  wires:
  Data Type Conversion1/1 -> ErrorToPower2/1(u)
  ErrorChecks/1 -> Data Type Conversion1/1
  ErrorToPower2/1(e) -> ErrorValue/1

== system model_base_bros/Robot1/DataToEtherCAT/FTSensorError ==
  RobotBus : Inport
  AvoidAlgebraicLoop : Memory
  Bus Selector : BusSelector  OutputSignals=BusFTSensor.ForcesSensorSpace
  Constant : Constant  Value=RobotStruct.FTSensor.MaxAllowableForcesTorqueSensor
  Data Type Conversion1 : DataTypeConversion  OutDataTypeStr=boolean
  Detect Change : simulink/Logic and Bit Operations/Detect Change  vinit=0  InputProcessing=Inherited  OutDataTypeStr=boolean
  FTSensorLastError : Display
  LatchRising : LibraryFM/Utilities/LatchRising  ic=0
  MATLAB Function : MATLAB Function  TreatAsAtomicUnit=on
  ShowFTSensorErrorLatched : Display
  FTSensorError : Outport
  FTSensorErrorLatched : Outport  Port=2
  wires:
  Constant/1 -> MATLAB Function/2(MaxForcesTorques)
  MATLAB Function/1(e) -> Data Type Conversion1/1, FTSensorLastError/1
  LatchRising/1 -> ShowFTSensorErrorLatched/1, FTSensorErrorLatched/1
  AvoidAlgebraicLoop/1 -> Detect Change/1, LatchRising/1, FTSensorError/1
  Detect Change/1 -> LatchRising/Trigger
  RobotBus/1 -> Bus Selector/1
  Bus Selector/1 -> MATLAB Function/1(ForcesTorques)  "<ForcesSensorSpace>"
  Data Type Conversion1/1 -> AvoidAlgebraicLoop/1

== system model_base_bros/Robot1/DataToEtherCAT/WorkspacePositionGuard ==
  note: Check internal angles
  note: Check whether endpoint position is within the predefined workspace
      | (ellipse)
  note: Check for singularity of joint configuration by checking
      | the condition number. When it exceeds a certain value, go to a safe mode
      | For now, this means disabling the actuators.
      | Note that the boundaries set using admittance should prohibit this from happening.
      | However, if sometjhing really goes wrong, this is a safe guard
  BusRobot : Inport
  StateSystem : Inport  Port=2
  AvoidAlgebraicLoop : Memory
  Bus Selector : BusSelector  OutputSignals=xOpSpace.x,xOpSpace.conditioning,qJointSpace.q_all
  CheckInternalAngles : MATLAB Function  TreatAsAtomicUnit=on
  Compare To Constant : simulink/Logic and Bit Operations/Compare To Constant  relop=>  const=4  OutDataTypeStr=boolean
  Compare To Constant1 : simulink/Logic and Bit Operations/Compare To Constant  relop=>=  const=2.75  OutDataTypeStr=boolean
  Data Type Conversion1 : DataTypeConversion  OutDataTypeStr=boolean
  Data Type Conversion2 : DataTypeConversion  Commented=through  OutDataTypeStr=int32
  Data Type Conversion4 : DataTypeConversion  OutDataTypeStr=boolean
  Detect Change : simulink/Logic and Bit Operations/Detect Change  vinit=0  InputProcessing=Inherited  OutDataTypeStr=boolean
  EndpointPositionGuard : MATLAB Function  TreatAsAtomicUnit=on
  LatchRising : LibraryFM/Utilities/LatchRising  ic=0
  Logical Operator : Logic  Operator=OR  AllPortsSameDT=off  OutDataTypeStr=boolean
  Mux : Mux  Inputs=2
  ShowWorkspaceErrorLatched : Display
  WorkspaceLastError : Display
  WorkspaceError : Outport
  WorkspaceErrorLatched : Outport  Port=2
  wires:
  BusRobot/1 -> Bus Selector/1
  Bus Selector/1 -> EndpointPositionGuard/2(xe)  "<x>"
  LatchRising/1 -> Data Type Conversion2/1
  EndpointPositionGuard/1(error) -> Data Type Conversion1/1
  Mux/1 -> AvoidAlgebraicLoop/1, WorkspaceLastError/1
  Detect Change/1 -> LatchRising/Trigger
  AvoidAlgebraicLoop/1 -> WorkspaceError/1, Detect Change/1, LatchRising/1
  Compare To Constant/1 -> EndpointPositionGuard/1(correctState)
  Bus Selector/2 -> Compare To Constant1/1  "<conditioning>"
  StateSystem/1 -> Compare To Constant/1
  Data Type Conversion2/1 -> WorkspaceErrorLatched/1, ShowWorkspaceErrorLatched/1
  CheckInternalAngles/1(angleError) -> Data Type Conversion4/1
  Bus Selector/3 -> CheckInternalAngles/1(theta)  "<q_all>"
  Data Type Conversion4/1 -> Mux/2
  Logical Operator/1 -> Mux/1
  Data Type Conversion1/1 -> Logical Operator/1
  Compare To Constant1/1 -> Logical Operator/2

== system model_base_bros/Robot2/Controller_PD/PD + nonlin (op space) ==
  x_ref : Inport
  xdot_ref : Inport  Port=2
  xddot_ref : Inport  Port=3
  RobotBus : Inport  Port=4
  systemState : Inport  Port=5
  Bus Creator : BusCreator  Inputs=2
  Bus Selector : BusSelector  OutputSignals=xOpSpace.x,xOpSpace.xdot,xOpSpace.x_AbsEnc,xOpSpace.xdot_AbsEnc,xOpSpace.J,xOpSpace.Jdot,qJointSpace.qdot_IncEnc
  DesiredTorque_PID : Display
  Gain : Gain  Gain=0
  Kd : Gain  Gain=15
  Kd1 : Gain  Gain=0
  Kd2 : Gain  Gain=5
  Kp : Gain  Gain=1500
  Sum{,2,4..5} (4 alike) : Sum  Inputs=|+-
  Sum1 : Sum  Inputs=|++
  Sum3 : Sum  Inputs=++++
  Terminator : Terminator
  Terminator1 : Terminator
  invJ1 : MATLAB Function  TreatAsAtomicUnit=on
  nonlinear compensation : MATLAB Function  TreatAsAtomicUnit=on
  JointTorqueDes_Nm : Outport
  ToLogger : Outport  Port=2
  wires:
  nonlinear compensation/1(tau) -> Gain/1, Bus Creator/2  "tau_nlcomp"
  invJ1/1(y) -> Sum1/1, Bus Creator/1  "tau_y"
  Bus Selector/1 -> Sum/2  "<x>"
  x_ref/1 -> Sum/1, Sum4/1  "q_ref"
  Sum/1 -> Kp/1  "e_p"
  xdot_ref/1 -> Sum5/1, Sum2/1  "qdot_ref"
  Sum2/1 -> Kd/1  "e_d"
  Sum1/1 -> JointTorqueDes_Nm/1, DesiredTorque_PID/1
  systemState/1 -> Terminator/1
  Bus Creator/1 -> ToLogger/1  "ToLoggerPD"
  Gain/1 -> Sum1/2
  Bus Selector/2 -> Sum2/2  "<xdot>"
  Bus Selector/6 -> nonlinear compensation/2(Jdot)  "<Jdot>"
  Bus Selector/5 -> nonlinear compensation/1(J), invJ1/2(J)  "<J>"
  RobotBus/1 -> Bus Selector/1
  Sum4/1 -> Kd1/1
  Sum5/1 -> Kd2/1
  xddot_ref/1 -> Terminator1/1  "qddot_ref"
  Bus Selector/3 -> Sum4/2  "<x_AbsEnc>"
  Bus Selector/4 -> Sum5/2  "<xdot_AbsEnc>"
  Kd/1 -> Sum3/2
  Kp/1 -> Sum3/1
  Sum3/1 -> invJ1/1(x)
  Kd1/1 -> Sum3/3
  Kd2/1 -> Sum3/4
  Bus Selector/7 -> nonlinear compensation/3(qdot)  "<qdot_IncEnc>"

== system model_base_bros/Robot2/Controller_PD/at home ==
  note: The velocity and acceleration references are set to [0;0] for stability.
  HomePosition : Inport
  Action Port : ActionPort  InitializeStates=reset  ActionType=case
  Constant : Constant
  Constant2 : Constant  Value=[0;0]
  Constant4 : Constant  Value=[0;0]
  HoldFirstSampleOnEnable : Subsystem
  x_ref : Outport  InitialOutput=[0;0]
  xdot_ref : Outport  Port=2  InitialOutput=[0;0]
  xddot_ref : Outport  Port=3  InitialOutput=[0;0]
  wires:
  Constant2/1 -> xdot_ref/1
  HoldFirstSampleOnEnable/1(x0) -> x_ref/1
  Constant4/1 -> xddot_ref/1
  Constant/1 -> HoldFirstSampleOnEnable/Enable
  HomePosition/1 -> HoldFirstSampleOnEnable/1(x)

== system model_base_bros/Robot2/Controller_PD/default ==
  Action Port : ActionPort  InitializeStates=reset  ActionType=default
  Constant3 : Constant  Value=[0;0]
  JointTorqueDes_Nm : Outport  InitialOutput=[0;0]
  wires:
  Constant3/1 -> JointTorqueDes_Nm/1

== system model_base_bros/Robot2/Controller_PD/homing - active ==
  note: The velocity and acceleration references are set to [0;0] for stability.
  HomePosition : Inport
  RobotBus : Inport  Port=2
  Action Port : ActionPort  InitializeStates=reset  ActionType=case
  Bus Selector : BusSelector  OutputSignals=xOpSpace.x
  Constant1 : Constant
  Constant2 : Constant  Value=[0;0]
  Constant4 : Constant  Value=[0;0]
  CrossFade : VariousBlocksLibrary/Various/CrossFade
  Cycloid : VariousBlocksLibrary/Various/Cycloid
  Rate Limiter : RateLimiter  RisingSlewLimit=0.1  FallingSlewLimit=-0.2  SampleTimeMode=inherited
  x_ref : Outport  InitialOutput=[0;0]
  xdot_ref : Outport  Port=2  InitialOutput=[0;0]
  xddot_ref : Outport  Port=3  InitialOutput=[0;0]
  wires:
  Constant2/1 -> xdot_ref/1
  Bus Selector/1 -> CrossFade/1  "<x>"
  RobotBus/1 -> Bus Selector/1
  HomePosition/1 -> CrossFade/2
  Cycloid/1 -> CrossFade/3
  Rate Limiter/1 -> Cycloid/1
  Constant1/1 -> Rate Limiter/1
  CrossFade/1 -> x_ref/1
  Constant4/1 -> xddot_ref/1

== system model_base_bros/Robot2/Controller_PD/idle (no torque) ==
  Action Port : ActionPort  InitializeStates=reset  ActionType=case
  Constant3 : Constant  Value=[0;0]
  JointTorqueDes_Nm : Outport  InitialOutput=[0;0]
  wires:
  Constant3/1 -> JointTorqueDes_Nm/1

== system model_base_bros/Robot2/Controller_PD/run ==
  x_ref_in : Inport
  xdot_ref_in : Inport  Port=2
  xddot_ref_in : Inport  Port=3
  Action Port : ActionPort  InitializeStates=reset  ActionType=case
  x_ref : Outport  InitialOutput=[0;0]
  xdot_ref : Outport  Port=2  InitialOutput=[0;0]
  xddot_ref : Outport  Port=3  InitialOutput=[0;0]
  wires:
  xdot_ref_in/1 -> xdot_ref/1
  xddot_ref_in/1 -> xddot_ref/1
  x_ref_in/1 -> x_ref/1

== system model_base_bros/Robot2/DataFromEtherCAT/Calculate Arrange Joint and Op Space ==
  note: Here all angles of the parallel mechanism are calculated
      | based on the endpoint position, though this may still lead to incorrect
      | estimations of the internal angles (e.g. it is possible that on of the elbows
      | has gone through a singular position already). So perhaps I should also include
      | a different way of calculating the internal angles
  BusActuators : Inport
  Bus Creator1 : BusCreator  Inputs=9
  Bus Creator2 : BusCreator  Inputs=6
  Bus Selector1 : BusSelector  OutputSignals=BusActuator1.JointPosition_AbsEnc_rad,BusActuator2.JointPosition_AbsEnc_rad,BusActuator1.JointVelocity_AbsEnc_rads,BusActuator2.JointVelocity_AbsEnc_rads
  Bus Selector2 : BusSelector  OutputSignals=BusActuator1.JointPosition_IncEnc_rad,BusActuator2.JointPosition_IncEnc_rad,BusActuator1.JointVelocity_IncEnc_rads,BusActuator2.JointVelocity_IncEnc_rads
  Bus Selector3 : BusSelector  OutputSignals=BusActuator1.JointTorque_Act_Nm,BusActuator2.JointTorque_Act_Nm
  Condition number : MATLAB Function  TreatAsAtomicUnit=on
  Ground : Ground
  Ground1 : Ground
  IK all joints : MATLAB Function  TreatAsAtomicUnit=on
  Mux{,1..4} (5 alike) : Mux  Inputs=2
  Terminator1 : Terminator
  Terminator2 : Terminator
  forward kinematics : Subsystem
  forward kinematics1 : Subsystem
  xOpSpace : Outport
  qJointSpace : Outport  Port=2
  wires:
  forward kinematics/5(Jdot) -> Bus Creator1/4  "Jdot"
  forward kinematics/3(xddot) -> Terminator1/1
  forward kinematics/2(xdot) -> Bus Creator1/2  "xdot"
  forward kinematics/1(x) -> IK all joints/1(x), Bus Creator1/1  "x"
  Bus Creator1/1 -> xOpSpace/1  "xOpSpace"
  forward kinematics/4(J) -> Condition number/1(J), Bus Creator1/3  "J"
  Ground/1 -> forward kinematics/3(JointAcceleration_rads2)
  Bus Creator2/1 -> qJointSpace/1  "qJointSpace"
  BusActuators/1 -> Bus Selector1/1, Bus Selector3/1, Bus Selector2/1
  Bus Selector2/1 -> Mux/1  "<JointPosition_IncEnc_rad>"
  Bus Selector2/2 -> Mux/2  "<JointPosition_IncEnc_rad>"
  Bus Selector2/3 -> Mux1/1  "<JointVelocity_IncEnc_rads>"
  Bus Selector2/4 -> Mux1/2  "<JointVelocity_IncEnc_rads>"
  Mux1/1 -> Bus Creator2/3, forward kinematics/2(JointVelocity_rads)  "qdot_IncEnc"
  Mux/1 -> forward kinematics/1(JointPosition_rad), Bus Creator2/2  "q_IncEnc"
  IK all joints/1(q_all) -> Bus Creator2/6  "q_all"
  Condition number/1(C) -> Bus Creator1/5  "conditioning"
  Bus Selector1/4 -> Mux3/2  "<JointVelocity_AbsEnc_rads>"
  Bus Selector1/3 -> Mux3/1  "<JointVelocity_AbsEnc_rads>"
  Bus Selector1/2 -> Mux2/2  "<JointPosition_AbsEnc_rad>"
  Bus Selector1/1 -> Mux2/1  "<JointPosition_AbsEnc_rad>"
  forward kinematics1/3(xddot) -> Terminator2/1
  Ground1/1 -> forward kinematics1/3(JointAcceleration_rads2)
  Mux2/1 -> Bus Creator2/4, forward kinematics1/1(JointPosition_rad)  "q_AbsEnc"
  Mux3/1 -> Bus Creator2/5, forward kinematics1/2(JointVelocity_rads)  "qdot_AbsEnc"
  forward kinematics1/2(xdot) -> Bus Creator1/7  "xdot_AbsEnc"
  forward kinematics1/1(x) -> Bus Creator1/6  "x_AbsEnc"
  forward kinematics1/4(J) -> Bus Creator1/8  "J_AbsEnc"
  forward kinematics1/5(Jdot) -> Bus Creator1/9  "Jdot_AbsEnc"
  Bus Selector3/1 -> Mux4/1  "<JointTorque_Act_Nm>"
  Bus Selector3/2 -> Mux4/2  "<JointTorque_Act_Nm>"
  Mux4/1 -> Bus Creator2/1  "JointTorque_Nm"

== system model_base_bros/Robot2/DataFromEtherCAT/FTSensor_K6D27 ==
  qJointSpace : Inport
  CorrectSensorOffset : Inport  Port=2
  AI1_ch0 : Inport  Port=3
  AI2_ch1 : Inport  Port=4
  AI3_ch2 : Inport  Port=5
  AI4_ch3 : Inport  Port=6
  AI5_ch4 : Inport  Port=7
  AI6_ch5 : Inport  Port=8
  Bus Creator : BusCreator  Inputs=3
  Bus Selector : BusSelector  OutputSignals=q_all
  Constant : Constant  Value=FTSensorStruct.TransformationMatrixSide
  CorrectOffset : MATLAB Function  TreatAsAtomicUnit=on
  Data Type Conversion{,1..5} (6 alike) : DataTypeConversion  OutDataTypeStr=double
  Detect Increase : simulink/Logic and Bit Operations/Detect Increase  vinit=0.0  InputProcessing=Inherited  OutDataTypeStr=boolean
  Mux : Mux  Inputs=6
  Selector : Selector  InputPortWidth=6  IndexOptions=Index vector (dialog)  Indices=[1 2]  OutputSizes=1
  SensorToOperationalSpace : MATLAB Function  TreatAsAtomicUnit=on
  Terminator : Terminator
  force (op space) : Display
  force (sensor space) : Display
  spikefilter : Subsystem
  Bus_FTSensor : Outport
  wires:
  Constant/1 -> SensorToOperationalSpace/3(transmatside)
  Bus Creator/1 -> Bus_FTSensor/1  "BusFTSensor"
  SensorToOperationalSpace/1(FTOpSpace) -> Selector/1, force (op space)/1, Bus Creator/1  "ForcesOpSpace"
  CorrectOffset/1(u_out) -> spikefilter/1(in)  "ForcesSensorSpace"
  CorrectOffset/2(corrected) -> Terminator/1
  AI3_ch2/1 -> Data Type Conversion2/1
  AI4_ch3/1 -> Data Type Conversion3/1
  AI5_ch4/1 -> Data Type Conversion4/1
  AI6_ch5/1 -> Data Type Conversion5/1
  Detect Increase/1 -> CorrectOffset/2(reset)
  CorrectSensorOffset/1 -> Detect Increase/1
  Mux/1 -> CorrectOffset/1(u_in)
  AI1_ch0/1 -> Data Type Conversion/1
  AI2_ch1/1 -> Data Type Conversion1/1
  qJointSpace/1 -> Bus Selector/1
  Bus Selector/1 -> SensorToOperationalSpace/1(q_all)  "<q_all>"
  Selector/1 -> Bus Creator/2  "FxFyOpSpace"
  Data Type Conversion/1 -> Mux/1
  Data Type Conversion1/1 -> Mux/2
  Data Type Conversion2/1 -> Mux/3
  Data Type Conversion3/1 -> Mux/4
  Data Type Conversion4/1 -> Mux/5
  Data Type Conversion5/1 -> Mux/6
  spikefilter/1(out) -> SensorToOperationalSpace/2(Fs), Bus Creator/3, force (sensor space)/1  "ForcesSensorSpace"

== system model_base_bros/Robot2/DataToEtherCAT/CreateSingleErrorValue1 ==
  ErrorChecks : Inport
  Data Type Conversion1 : DataTypeConversion  OutDataTypeStr=double
  ErrorToPower2 : MATLAB Function  TreatAsAtomicUnit=on
  ErrorValue : Outport
  wires:
  Data Type Conversion1/1 -> ErrorToPower2/1(u)
  ErrorChecks/1 -> Data Type Conversion1/1
  ErrorToPower2/1(e) -> ErrorValue/1

== system model_base_bros/Robot2/DataToEtherCAT/CreateSingleErrorValue2 ==
  ErrorChecks : Inport
  Data Type Conversion1 : DataTypeConversion  OutDataTypeStr=double
  ErrorToPower2 : MATLAB Function  TreatAsAtomicUnit=on
  ErrorValue : Outport
  wires:
  Data Type Conversion1/1 -> ErrorToPower2/1(u)
  ErrorChecks/1 -> Data Type Conversion1/1
  ErrorToPower2/1(e) -> ErrorValue/1

== system model_base_bros/Robot2/DataToEtherCAT/FTSensorError ==
  RobotBus : Inport
  AvoidAlgebraicLoop : Memory
  Bus Selector : BusSelector  OutputSignals=BusFTSensor.ForcesSensorSpace
  Constant : Constant  Value=RobotStruct.FTSensor.MaxAllowableForcesTorqueSensor
  Data Type Conversion1 : DataTypeConversion  OutDataTypeStr=boolean
  Detect Change : simulink/Logic and Bit Operations/Detect Change  vinit=0  InputProcessing=Inherited  OutDataTypeStr=boolean
  FTSensorLastError : Display
  LatchRising : LibraryFM/Utilities/LatchRising  ic=0
  MATLAB Function : MATLAB Function  TreatAsAtomicUnit=on
  ShowFTSensorErrorLatched : Display
  FTSensorError : Outport
  FTSensorErrorLatched : Outport  Port=2
  wires:
  Constant/1 -> MATLAB Function/2(MaxForcesTorques)
  MATLAB Function/1(e) -> Data Type Conversion1/1, FTSensorLastError/1
  LatchRising/1 -> ShowFTSensorErrorLatched/1, FTSensorErrorLatched/1
  AvoidAlgebraicLoop/1 -> Detect Change/1, LatchRising/1, FTSensorError/1
  Detect Change/1 -> LatchRising/Trigger
  RobotBus/1 -> Bus Selector/1
  Bus Selector/1 -> MATLAB Function/1(ForcesTorques)  "<ForcesSensorSpace>"
  Data Type Conversion1/1 -> AvoidAlgebraicLoop/1
